simulink model "BMS_final"  (R2021a)
settings: Solver=VariableStepAuto  StartTime=0.0  StopTime=2000  RelTol=1e-3
undefined symbols (not defined in the file): Ion, Lithium
libraries: spsBatteryLib x26, spsCurrentMeasurementLib x1, spsMosfetLib x1, spsVoltageMeasurementLib x1, spsSeriesRLCBranchLib x1, spspowerguiLib x1
settings Model: Creator=msipc  LastModifiedBy=msipc

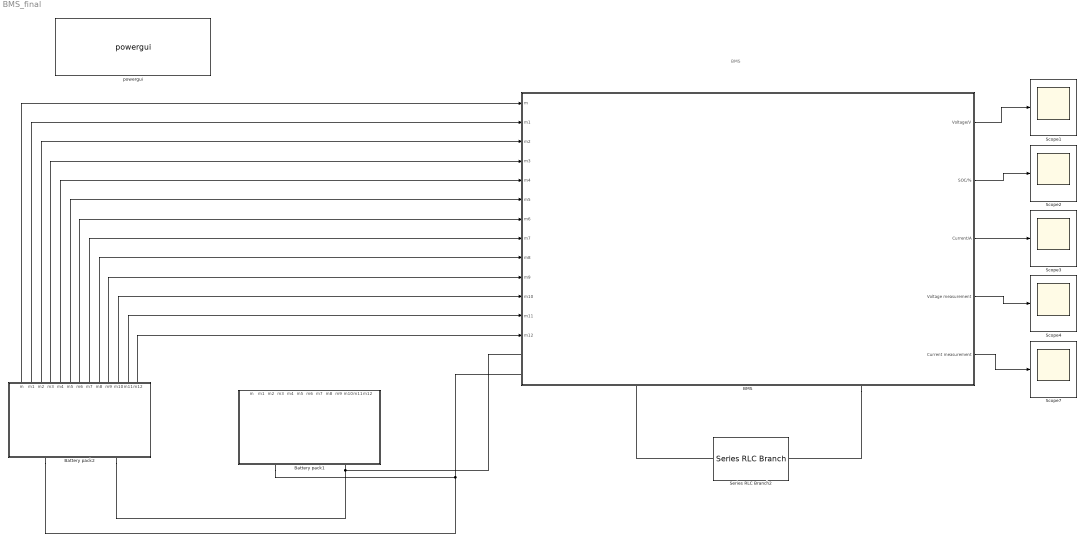
== system BMS_final ==
  note: BMS
  BMS : Subsystem
      settings: PortSchema="{\"entries\":[{\"content\":{\"sides\":[{\"content\":{\"connectorIds\":[\"In1\",\"In2\",\"In3\",\"In4\",\"In5\",\"In6\",\"In7\",\"In8\",\"In9\",\"In10\",\"In11\",\"In12\",\"In13\",\"LConn1\",\"LConn2\"]},\"type\":\"ConnectorPlacement.EquallySpacedRectSide\",\"uuid\":\"dd94a0c2-7f1a-48af-bd53-36167d1f7532\"},{\"content\":{\"connectorIds\":[\"Out1\",\"Out2\",\"Out3\",\"Out4\",\"Out5\"],\"side\":\"RIGHT\"},\"type\":\"ConnectorPlacement.EquallySpacedRectSide\",\"uuid\":\"c08fe822-2b26-4f55-837a-808c5fcf1752\"},{\"content\":{\"connectorIds\":[],\"side\":\"TOP\"},\"type\":\"ConnectorPlacement.EquallySpacedRectSide\",\"uuid\":\"095bc00f-5241-4436-9c7a-20955f305706\"},{\"content\":{\"connectorIds\":[\"RConn1\",\"RConn2\"],\"side\":\"BOTTOM\"},\"type\":\"ConnectorPlacement.EquallySpacedRectSide\",\"uuid\":\"82e8aaac-5d89-4979-90f0-73b1a1fe5a1e\"}]},\"type\":\"ConnectorPlacement.EquallySpacedConnector\",\"uuid\":\"8a6a1581-9e2f-4562-a585-c5418e332f97\"}],\"packageUris\":[\"http://schema.mathworks.com/mf0/Connector/R2020b\"],\"version\":\"1.0\"}"
  Battery pack1 : Subsystem
  Battery pack2 : Subsystem
  Scope{1..4,7} (5 alike) : Scope
  Series RLC Branch2 : spsSeriesRLCBranchLib/Series RLC Branch  LConnTagsString=__new0  RConnTagsString=__new0  BranchType=R  Resistance=1000  Inductance=1e-3  SetiL0=off  InitialCurrent=0  Capacitance=1e-6  Setx0=off  InitialVoltage=0  Measurements=None
  powergui : spspowerguiLib/powergui  Priority=1  SimulationMode=Continuous  SampleTime=50e-6  frequency=60  Iterations=50  frequencyindice=0  Pbase=100e6  ErrMax=1e-4  UnitsV=kV  UnitsW=MW  buscounter=0  FunctionMessages=off  echomessages=off  EnableUseOfTLC=off  CurrentSourceSwitches=off  DisableSnubberDevices=off  DisableRonSwitches=off  DisableVfSwitches=off  DisplayEquations=off  AutomaticDiscreteSolvers=off  SolverType=Tustin/Backward Euler (TBE)  Interpol=off  ExternalGateDelay=off  methode=off  Ts=100  x0status=blocks  SPID=on  SwTol=0  HookPort=off  NonlinearTolerance=1e-4  nMaxIteration=100  ContinueOnMaxIteration=off  RestoreLinks=warning  ResistiveCurrentMeasurement=off  Frange=[0:2:500]  Ylog=off  Xlog=on  ShowGrid=off  save=off  variable=ZData  structure=0  ZoomFFT=off  StartTime=0.0  cycles=1  DisplayStyle=1  fundamental=60  FreqAxis=off  MaxFrequency=1000  frequencyindicesteady=1  RmsSteady=1  display=off
  wires:
  Battery pack2/1(m) -> BMS/1(m)
  Battery pack2/2(m1) -> BMS/2(m1)
  Battery pack2/3(m2) -> BMS/3(m2)
  Battery pack2/4(m3) -> BMS/4(m3)
  Battery pack2/5(m4) -> BMS/5(m4)
  Battery pack2/6(m5) -> BMS/6(m5)
  Battery pack2/7(m6) -> BMS/7(m6)
  Battery pack2/8(m7) -> BMS/8(m7)
  Battery pack2/9(m8) -> BMS/9(m8)
  Battery pack2/10(m9) -> BMS/10(m9)
  Battery pack2/11(m10) -> BMS/11(m10)
  Battery pack2/12(m11) -> BMS/12(m11)
  Battery pack2/13(m12) -> BMS/13(m12)
  BMS/2(SOC/%) -> Scope2/1
  BMS/1(Voltage/V) -> Scope1/1
  BMS/3(Current/A) -> Scope3/1
  BMS/4(Voltage measurement) -> Scope4/1
  BMS/5(Current measurement) -> Scope7/1
  connections:
  Battery pack2/LConn1 -- Battery pack1/LConn1 -- BMS/LConn2
  Battery pack2/LConn2 -- BMS/LConn1 -- Battery pack1/LConn2
  BMS/RConn2 -- Series RLC Branch2/RConn1
  Series RLC Branch2/LConn1 -- BMS/RConn1

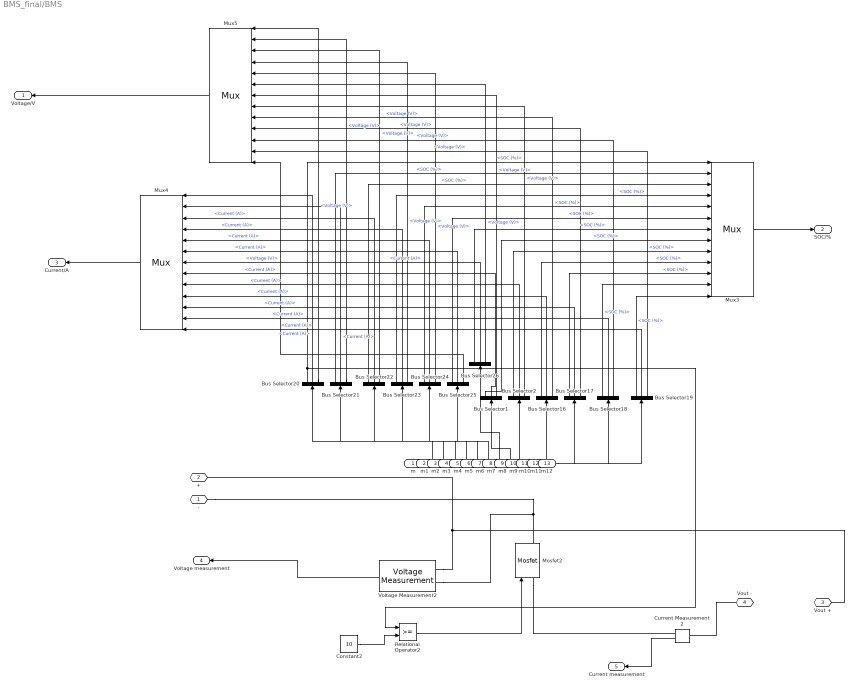
== system BMS_final/BMS ==
  m : Inport
  m1 : Inport  Port=2
  m2 : Inport  Port=3
  m3 : Inport  Port=4
  m4 : Inport  Port=5
  m5 : Inport  Port=6
  m6 : Inport  Port=7
  m7 : Inport  Port=8
  m8 : Inport  Port=9
  m9 : Inport  Port=10
  m10 : Inport  Port=11
  m11 : Inport  Port=12
  m12 : Inport  Port=13
  Bus Selector{1..2,16..26} (13 alike) : BusSelector  OutputSignals=SOC (%),Current (A),Voltage (V)
  Constant2 : Constant  Value=10
  Current Measurement2 : spsCurrentMeasurementLib/Current Measurement  PhasorSimulation=off  OutputType=Complex  PSBequivalent=0
  Mosfet2 : spsMosfetLib/Mosfet  Ron=0.1  Lon=0  Rd=0.01  Vfd=0  IC=0  Rs=1e5  Cs=inf  Measurements=on
  Mux3 : Mux  Inputs=13
  Mux4 : Mux  Inputs=13
  Mux5 : Mux  Inputs=13
  Relational Operator2 : RelationalOperator  OutDataTypeStr=boolean  RndMeth=Simplest
  Voltage Measurement2 : spsVoltageMeasurementLib/Voltage Measurement  PhasorSimulation=off  OutputType=Complex  PSBequivalent=0
  - : PMIOPort  Side=Left
  + : PMIOPort  Port=2  Side=Left
  "Vout + " : PMIOPort  Port=3  Side=Right
  Vout - : PMIOPort  Port=4  Side=Right
  Voltage/V : Outport
  SOC/% : Outport  Port=2
  Current/A : Outport  Port=3
  Voltage measurement : Outport  Port=4
  Current measurement : Outport  Port=5
  wires:
  Bus Selector25/3 -> Mux5/13  "<Voltage (V)>"
  Bus Selector1/3 -> Mux5/7  "<Voltage (V)>"
  Bus Selector22/3 -> Mux5/3  "<Voltage (V)>"
  Bus Selector18/3 -> Mux5/11  "<Voltage (V)>"
  Bus Selector17/3 -> Mux5/10  "<Voltage (V)>"
  m/1 -> Bus Selector20/1
  Bus Selector26/3 -> Mux5/6  "<Voltage (V)>"
  m1/1 -> Bus Selector21/1
  Bus Selector18/2 -> Mux4/12  "<Current (A)>"
  Bus Selector16/3 -> Mux5/9  "<Voltage (V)>"
  Mux5/1 -> Voltage/V/1
  Bus Selector2/3 -> Mux5/8  "<Voltage (V)>"
  m9/1 -> Bus Selector16/1
  Bus Selector24/3 -> Mux5/5  "<Voltage (V)>"
  m2/1 -> Bus Selector22/1
  Relational Operator2/1 -> Mosfet2/1
  Mux3/1 -> SOC/%/1
  Bus Selector18/1 -> Mux3/12  "<SOC (%)>"
  m6/1 -> Bus Selector26/1
  Bus Selector23/3 -> Mux5/4  "<Voltage (V)>"
  Bus Selector20/3 -> Mux5/1  "<Voltage (V)>"
  Bus Selector20/1 -> Relational Operator2/1, Mux3/1  "<SOC (%)>"
  Bus Selector23/1 -> Mux3/4  "<SOC (%)>"
  Bus Selector17/1 -> Mux3/11  "<SOC (%)>"
  Bus Selector21/3 -> Mux5/2  "<Voltage (V)>"
  Bus Selector16/2 -> Mux4/10  "<Current (A)>"
  Bus Selector19/2 -> Mux4/13  "<Current (A)>"
  Bus Selector19/3 -> Mux5/12  "<Voltage (V)>"
  Bus Selector17/2 -> Mux4/11  "<Current (A)>"
  Bus Selector1/2 -> Mux4/8  "<Current (A)>"
  Bus Selector2/2 -> Mux4/9  "<Current (A)>"
  Bus Selector26/2 -> Mux4/7  "<Current (A)>"
  Current Measurement2/1 -> Current measurement/1
  Bus Selector25/2 -> Mux4/6  "<Current (A)>"
  Bus Selector24/2 -> Mux4/5  "<Current (A)>"
  Bus Selector23/2 -> Mux4/4  "<Current (A)>"
  Bus Selector2/1 -> Mux3/9  "<SOC (%)>"
  Bus Selector22/2 -> Mux4/3  "<Current (A)>"
  m11/1 -> Bus Selector18/1
  Bus Selector20/2 -> Mux4/1  "<Current (A)>"
  Bus Selector21/2 -> Mux4/2  "<Current (A)>"
  Bus Selector22/1 -> Mux3/3  "<SOC (%)>"
  Bus Selector19/1 -> Mux3/13  "<SOC (%)>"
  m4/1 -> Bus Selector24/1
  Bus Selector16/1 -> Mux3/10  "<SOC (%)>"
  Bus Selector26/1 -> Mux3/7  "<SOC (%)>"
  Voltage Measurement2/1 -> Voltage measurement/1
  Bus Selector1/1 -> Mux3/8  "<SOC (%)>"
  Bus Selector25/1 -> Mux3/6  "<SOC (%)>"
  Constant2/1 -> Relational Operator2/2
  m7/1 -> Bus Selector1/1
  Bus Selector24/1 -> Mux3/5  "<SOC (%)>"
  Bus Selector21/1 -> Mux3/2  "<SOC (%)>"
  m5/1 -> Bus Selector25/1
  m3/1 -> Bus Selector23/1
  Mux4/1 -> Current/A/1
  m10/1 -> Bus Selector17/1
  m12/1 -> Bus Selector19/1
  m8/1 -> Bus Selector2/1
  connections:
  Vout -/RConn1 -- Current Measurement2/LConn1
  Voltage Measurement2/LConn2 -- -/RConn1 -- Mosfet2/RConn1
  Voltage Measurement2/LConn1 -- "Vout + "/RConn1 -- +/RConn1
  Mosfet2/LConn1 -- Current Measurement2/RConn1

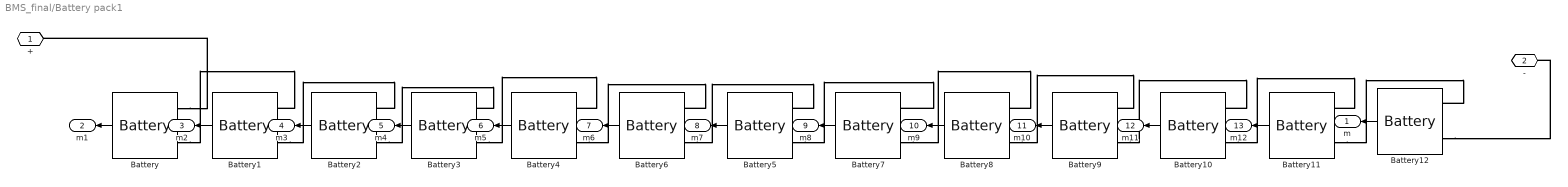
== system BMS_final/Battery pack1 ==
  Battery{,1..12} (13 alike) : spsBatteryLib/Battery  BatType=Lithium-Ion  ShowTempParam=off  ThermalPreset=no  ShowAgeParam=off  NomV=3.6  NomQ=2.5  SOC=100  Batt_Tr=5  PresetModel=on  MaxQ=2.5  MinV=2.7  FullV=4.1904  Dis_rate=1.087  R=0.0144  Normal_OP=2.2609  expZone="[3.8894     0.12283]"  current=[6.5 13 32.5]  Units=Time  Tci=20  NomT=20  T2=-30  MaxQ2=4.8  FullV2=7.1  Normal_OP2=5.655  expZone2="[6.58           1]"  Rca=0.6  ti=2000  Dp=0  Neq0=0  Tsim=1e6  Ta1=25  Qeol=5.4*0.9  Reol=0.013333*1.2  Char_age=[2.3478, 3]  Dis_age=[2.3478, 10]  N1=1500  N2=10500  N3=1000  N4=1400  Ta2=45  N5=950
  + : PMIOPort  Side=Left
  - : PMIOPort  Port=2  Side=Left
  m : Outport
  m1 : Outport  Port=2
  m2 : Outport  Port=3
  m3 : Outport  Port=4
  m4 : Outport  Port=5
  m5 : Outport  Port=6
  m6 : Outport  Port=7
  m7 : Outport  Port=8
  m8 : Outport  Port=9
  m9 : Outport  Port=10
  m10 : Outport  Port=11
  m11 : Outport  Port=12
  m12 : Outport  Port=13
  wires:
  Battery/1 -> m1/1
  Battery7/1 -> m8/1
  Battery9/1 -> m10/1
  Battery2/1 -> m3/1
  Battery3/1 -> m4/1
  Battery8/1 -> m9/1
  Battery1/1 -> m2/1
  Battery12/1 -> m/1
  Battery4/1 -> m5/1
  Battery6/1 -> m6/1
  Battery5/1 -> m7/1
  Battery11/1 -> m12/1
  Battery10/1 -> m11/1
  connections:
  Battery4/LConn2 -- Battery6/LConn1
  Battery2/LConn2 -- Battery3/LConn1
  Battery/LConn2 -- Battery1/LConn1
  Battery3/LConn2 -- Battery4/LConn1
  Battery9/LConn2 -- Battery10/LConn1
  Battery8/LConn2 -- Battery9/LConn1
  Battery1/LConn2 -- Battery2/LConn1
  Battery11/LConn2 -- Battery12/LConn1
  Battery6/LConn2 -- Battery5/LConn1
  Battery7/LConn2 -- Battery8/LConn1
  Battery10/LConn2 -- Battery11/LConn1
  Battery5/LConn2 -- Battery7/LConn1
  Battery12/LConn2 -- -/RConn1
  Battery/LConn1 -- +/RConn1

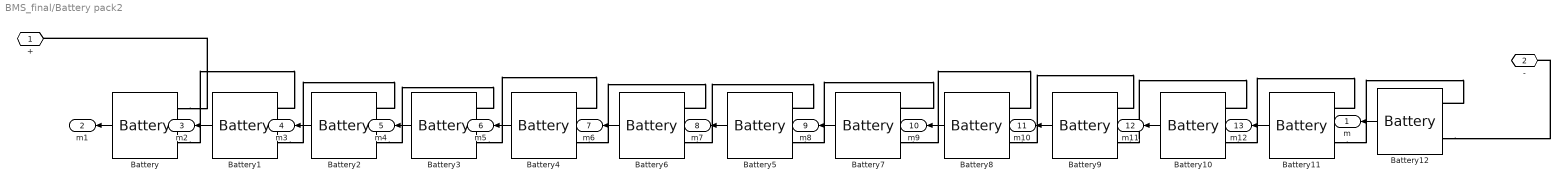
== system BMS_final/Battery pack2 ==
  Battery{,1..12} (13 alike) : spsBatteryLib/Battery  BatType=Lithium-Ion  ShowTempParam=off  ThermalPreset=no  ShowAgeParam=off  NomV=3.6  NomQ=2.5  SOC=100  Batt_Tr=5  PresetModel=on  MaxQ=2.5  MinV=2.7  FullV=4.1904  Dis_rate=1.087  R=0.0144  Normal_OP=2.2609  expZone="[3.8894     0.12283]"  current=[6.5 13 32.5]  Units=Time  Tci=20  NomT=20  T2=-30  MaxQ2=4.8  FullV2=7.1  Normal_OP2=5.655  expZone2="[6.58           1]"  Rca=0.6  ti=2000  Dp=0  Neq0=0  Tsim=1e6  Ta1=25  Qeol=5.4*0.9  Reol=0.013333*1.2  Char_age=[2.3478, 3]  Dis_age=[2.3478, 10]  N1=1500  N2=10500  N3=1000  N4=1400  Ta2=45  N5=950
  + : PMIOPort  Side=Left
  - : PMIOPort  Port=2  Side=Left
  m : Outport
  m1 : Outport  Port=2
  m2 : Outport  Port=3
  m3 : Outport  Port=4
  m4 : Outport  Port=5
  m5 : Outport  Port=6
  m6 : Outport  Port=7
  m7 : Outport  Port=8
  m8 : Outport  Port=9
  m9 : Outport  Port=10
  m10 : Outport  Port=11
  m11 : Outport  Port=12
  m12 : Outport  Port=13
  wires:
  Battery10/1 -> m11/1
  Battery11/1 -> m12/1
  Battery5/1 -> m7/1
  Battery6/1 -> m6/1
  Battery4/1 -> m5/1
  Battery12/1 -> m/1
  Battery1/1 -> m2/1
  Battery8/1 -> m9/1
  Battery3/1 -> m4/1
  Battery2/1 -> m3/1
  Battery9/1 -> m10/1
  Battery7/1 -> m8/1
  Battery/1 -> m1/1
  connections:
  Battery/LConn1 -- +/RConn1
  Battery12/LConn2 -- -/RConn1
  Battery5/LConn2 -- Battery7/LConn1
  Battery10/LConn2 -- Battery11/LConn1
  Battery7/LConn2 -- Battery8/LConn1
  Battery6/LConn2 -- Battery5/LConn1
  Battery11/LConn2 -- Battery12/LConn1
  Battery1/LConn2 -- Battery2/LConn1
  Battery8/LConn2 -- Battery9/LConn1
  Battery9/LConn2 -- Battery10/LConn1
  Battery3/LConn2 -- Battery4/LConn1
  Battery/LConn2 -- Battery1/LConn1
  Battery2/LConn2 -- Battery3/LConn1
  Battery4/LConn2 -- Battery6/LConn1
